simulink model "radice_cubica"  (R2017a)
settings: Solver=FixedStepDiscrete  StartTime=0.0  StopTime=inf  FixedStep=1  RelTol=1e-3
values from neighbouring files (symbols this model uses):
  a = 50    [radice.m]
  tol = 1e-3    (= 0.001)    [radice.m]
libraries: simulink x1
settings Model: Creator=Enrico Donato  LastModifiedBy=Enrico Donato

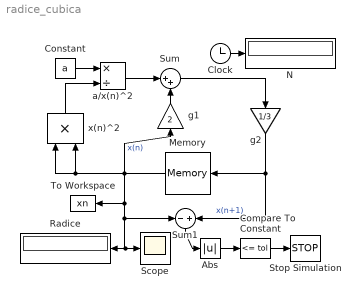
== system radice_cubica ==
  Abs : Abs
  Clock : Clock
  Compare To Constant : simulink/Logic and Bit Operations/Compare To Constant  relop=<=  const=tol  OutDataTypeStr=boolean
  Constant : Constant  Value=a
  Memory : Memory  X0=rand(1)
  N : Display
  Radice : Display
  Scope : Scope
  Stop Simulation : Stop
  Sum : Sum  Inputs=|++
  Sum1 : Sum  Inputs=-|+
  To Workspace : ToWorkspace  VariableName=xn  SampleTime=-1
      settings: Save2DSignal=2-D array (concatenate along first dimension)
  a/x(n)^2 : Product  Inputs=*/
  g1 : Gain  Gain=2
  g2 : Gain  Gain=1/3
  x(n)^2 : Product
  wires:
  g2/1 -> Sum1/2, Memory/1  "x(n+1)"
  Memory/1 -> g1/1, To Workspace/1, Sum1/1, Radice/1, Scope/1, x(n)^2/2, x(n)^2/1  "x(n)"
  x(n)^2/1 -> a/x(n)^2/2
  Constant/1 -> a/x(n)^2/1
  a/x(n)^2/1 -> Sum/1
  g1/1 -> Sum/2
  Sum/1 -> g2/1
  Sum1/1 -> Abs/1
  Abs/1 -> Compare To Constant/1
  Compare To Constant/1 -> Stop Simulation/1
  Clock/1 -> N/1
